simulink model "week2"  (R2020b)
settings: Solver=ode15s  StartTime=0.0  StopTime=0.2  RelTol=1e-3
values from neighbouring files (symbols this model uses):
  b = 3.5077E-6    [dd1.sldd]
  J = 3.2284E-6    [dd1.sldd]
  K = 0.0274    [dd1.sldd]
  L = 2.75E-6    [dd1.sldd]
  R = 4.0    [dd1.sldd]
settings Model: Creator=hp  LastModifiedBy=hp

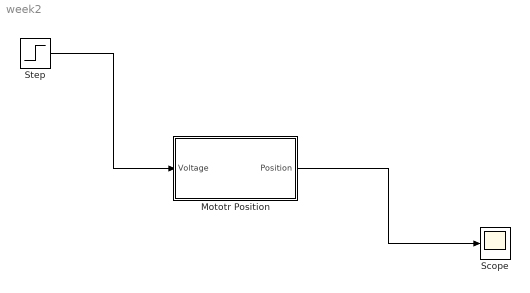
== system week2 ==
  Mototr Position : Subsystem
  Scope : Scope
  Step : Step  Time=0  SampleTime=0
  wires:
  Step/1 -> Mototr Position/1(Voltage)
  Mototr Position/1(Position) -> Scope/1

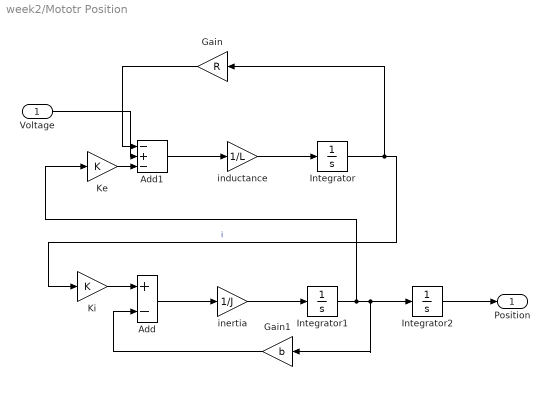
== system week2/Mototr Position ==
  Voltage : Inport
  Add : Sum  Inputs=+-
  Add1 : Sum  Inputs=-+-
  Gain : Gain  Gain=R
  Gain1 : Gain  Gain=b
  Integrator : Integrator
  Integrator1 : Integrator
  Integrator2 : Integrator
  Ke : Gain  Gain=K
  Ki : Gain  Gain=K
  inductance : Gain  Gain=1/L
  inertia : Gain  Gain=1/J
  Position : Outport
  wires:
  Add/1 -> inertia/1
  Integrator1/1 -> Ke/1, Gain1/1, Integrator2/1
  Gain1/1 -> Add/2
  Ke/1 -> Add1/3
  Integrator/1 -> Gain/1, Ki/1  "i"
  Gain/1 -> Add1/1
  Integrator2/1 -> Position/1
  inertia/1 -> Integrator1/1
  Ki/1 -> Add/1
  inductance/1 -> Integrator/1
  Voltage/1 -> Add1/2
  Add1/1 -> inductance/1
